simulink model "shuzisuoxfd"  (R2020b)
settings: Solver=VariableStepAuto  StartTime=0.0  StopTime=1000  RelTol=1e-3
libraries: dspsrcs4 x3, simulink x1, dspswit3 x1
settings Model: Creator=刘振宏  LastModifiedBy=LYX
settings DataIOCC: ReturnWorkspaceOutputs=off
settings DebuggingCC: ArithmeticOperatorsInVariantConditions=warning
settings SFSimCC: SimUseLocalCustomCode=off  CustomCodeUndefinedFunction=UseInterfaceOnly
settings RTWCC: RTWUseLocalCustomCode=off

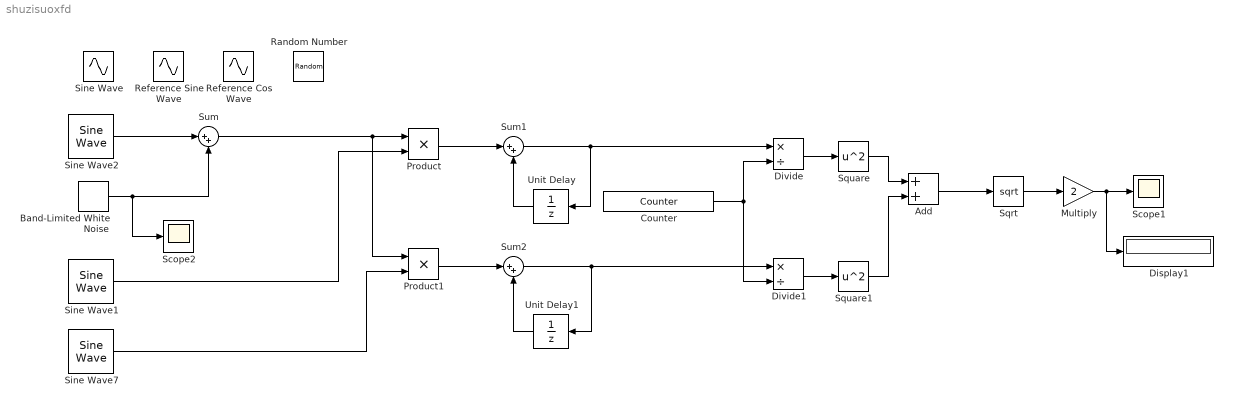
== system shuzisuoxfd ==
  Add : Sum
  Band-Limited White Noise : simulink/Sources/Band-Limited White Noise  Cov=[0.1*0.1*1/400]  Ts=1/240  seed=[23341]
  Counter : dspswit3/Counter  Direction=Up  CountEvent=Free running  CounterSize=32 bits  MaxCount=255  InitialCount=1  Output=Count  HitValue=32  ResetInput=off  SamplesPerFrame=1  Ts=1/240  CntDtype=single  HitDtype=Logical
  Display1 : Display
  Divide : Product  Inputs=*/
  Divide1 : Product  Inputs=*/
  Multiply : Gain  Gain=2
  Product : Product
  Product1 : Product
  Random Number : RandomNumber  Variance=4  SampleTime=0.05
  Reference Cos Wave : Sin  Amplitude=2  Frequency=2*pi  Phase=0.5*pi  SampleTime=0.05
  Reference Sine Wave : Sin  Amplitude=2  Frequency=2*pi  SampleTime=0.05
  Scope1 : Scope
  Scope2 : Scope
  Sine Wave : Sin  Amplitude=0.1  Frequency=2*pi  Phase=0.25*pi  SampleTime=0.05
  Sine Wave1 : dspsrcs4/Sine Wave  Amplitude=1  Frequency=20  Phase=0  SampleMode=Discrete  OutComplex=Real  CompMethod=Trigonometric fcn  TableSize=Speed  SampleTime=1/240  SamplesPerFrame=1  ResetState=Restart at time zero  OutputFrames=off  dataType=single  wordLen=16  udDataType=sfix(16)  fracBitsMode=Best precision  numFracBits=15  OutDataTypeStr=single  LastOutDataTypeStr=single
  Sine Wave2 : dspsrcs4/Sine Wave  Amplitude=0.001  Frequency=20  Phase=0  SampleMode=Discrete  OutComplex=Real  CompMethod=Trigonometric fcn  TableSize=Speed  SampleTime=1/240  SamplesPerFrame=1  ResetState=Restart at time zero  OutputFrames=off  dataType=single  wordLen=16  udDataType=sfix(16)  fracBitsMode=Best precision  numFracBits=15  OutDataTypeStr=single  LastOutDataTypeStr=single
  Sine Wave7 : dspsrcs4/Sine Wave  Amplitude=1  Frequency=20  Phase=pi/2  SampleMode=Discrete  OutComplex=Real  CompMethod=Trigonometric fcn  TableSize=Speed  SampleTime=1/240  SamplesPerFrame=1  ResetState=Restart at time zero  OutputFrames=off  dataType=single  wordLen=16  udDataType=sfix(16)  fracBitsMode=Best precision  numFracBits=15  OutDataTypeStr=single  LastOutDataTypeStr=single
  Sqrt : Sqrt  SaturateOnIntegerOverflow=on
  Square : Math  Operator=square  SignedPower=on  SaturateOnIntegerOverflow=on
  Square1 : Math  Operator=square  SignedPower=on  SaturateOnIntegerOverflow=on
  Sum : Sum  Inputs=|++
  Sum1 : Sum  Inputs=|++
  Sum2 : Sum  Inputs=|++
  Unit Delay : UnitDelay  SampleTime=-1  HasFrameUpgradeWarning=on
  Unit Delay1 : UnitDelay  SampleTime=-1  HasFrameUpgradeWarning=on
  wires:
  Sine Wave2/1 -> Sum/1
  Band-Limited White Noise/1 -> Scope2/1, Sum/2
  Sine Wave1/1 -> Product/2
  Sine Wave7/1 -> Product1/2
  Product/1 -> Sum1/1
  Unit Delay/1 -> Sum1/2
  Sum1/1 -> Unit Delay/1, Divide/1
  Counter/1 -> Divide1/2, Divide/2
  Product1/1 -> Sum2/1
  Sum2/1 -> Divide1/1, Unit Delay1/1
  Unit Delay1/1 -> Sum2/2
  Divide/1 -> Square/1
  Divide1/1 -> Square1/1
  Square/1 -> Add/1
  Square1/1 -> Add/2
  Add/1 -> Sqrt/1
  Sum/1 -> Product1/1, Product/1
  Sqrt/1 -> Multiply/1
  Multiply/1 -> Display1/1, Scope1/1
